simulink model "simulink_model"  (R2015a)
settings: Solver=ode3  StartTime=0.0  StopTime=20  RelTol=1e-3
undefined symbols (not defined in the file or in its folder): MIO, National_Instruments, PCI
libraries: sldrtlib x3, simulink x1
settings Model: SimulationMode=external  ExtModeTrigDuration=30001  Creator=Alunos  LastModifiedBy=Alunos
settings HardwareCC: ProdIntDivRoundTo=Zero  ProdEndianess=LittleEndian  ProdHWDeviceType=Intel->x86/Pentium  TargetIntDivRoundTo=Zero  TargetEndianess=LittleEndian  TargetHWDeviceType=Intel->x86/Pentium
settings RTWCC: SystemTargetFile=rtwin.tlc  TemplateMakefile=rtwin.tmf  Description=Simulink Desktop Real-Time  RTWCompilerOptimization=on
settings CodeAppCC: MaxIdLength=95
settings RTWinTargetCC: TargetPreCompLibLocation=C:\Program Files\MATLAB\R2015a\toolbox\sldrt\lib\win32

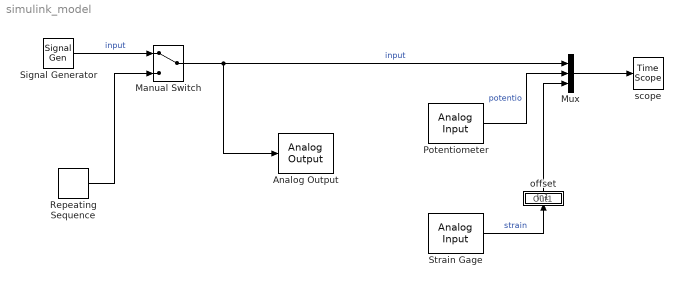
== system simulink_model ==
  Analog Output : sldrtlib/Analog Output  SampleTime=0.001  MaxMissedTicks=10  ShowMissedTicks=off  YieldWhenWaiting=off  DrvName=National_Instruments/PCI-MIO-16E-4  DrvAddress=4294967295  DrvOptions=[0 0 0 0 0 0]  Channels=1  RangeMode=1  VoltRange=1  InitialValue=0  FinalValue=0
      settings: AttributesFormatString=National Instruments\nPCI-MIO-16E-4 [auto]
  Manual Switch : ManualSwitch
  Mux : Mux  Inputs=3
  Potentiometer : sldrtlib/Analog Input  SampleTime=0.001  MaxMissedTicks=10  ShowMissedTicks=off  YieldWhenWaiting=off  DrvName=National_Instruments/PCI-MIO-16E-4  DrvAddress=4294967295  DrvOptions=[0 0 0 0 0 0]  Channels=1  RangeMode=1  VoltRange=1  DataType=1
      settings: AttributesFormatString=National Instruments\nPCI-MIO-16E-4 [auto]
  Repeating Sequence : simulink/Sources/Repeating Sequence  rep_seq_t=[0 0.9999 1 1.9999 2 2.9999 3 4]  rep_seq_y=[1 1 0 0 -1 -1 0 0]
  Signal Generator : SignalGenerator  WaveForm=square
  Strain Gage : sldrtlib/Analog Input  SampleTime=0.001  MaxMissedTicks=10  ShowMissedTicks=off  YieldWhenWaiting=off  DrvName=National_Instruments/PCI-MIO-16E-4  DrvAddress=4294967295  DrvOptions=[0 0 0 0 0 0]  Channels=2  RangeMode=1  VoltRange=1  DataType=1
      settings: AttributesFormatString=National Instruments\nPCI-MIO-16E-4 [auto]
  offset : Subsystem
  scope : TimeScope
  wires:
  Mux/1 -> scope/1
  Potentiometer/1 -> Mux/2  "potentio"
  Signal Generator/1 -> Manual Switch/1  "input"
  Manual Switch/1 -> Analog Output/1, Mux/1  "input"
  Repeating Sequence/1 -> Manual Switch/2
  Strain Gage/1 -> offset/1(In1)  "strain"
  offset/1(Out1) -> Mux/3

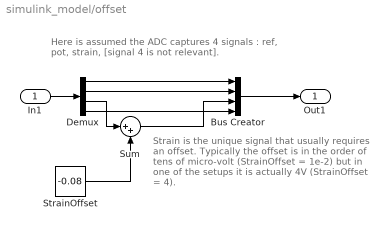
== system simulink_model/offset ==
  note: Strain is the unique signal that usually requires an offset. Typically the offset is in the order of tens of micro-volt (StrainOffset = 1e-2) but in one of the setups it is actually 4V (StrainOffset = 4).
  note: Here is assumed the ADC captures 4 signals :
      | ref, pot, strain, [signal 4 is not relevant].
  In1 : Inport
  Bus Creator : BusCreator
  Demux : Demux
  StrainOffset : Constant  Value=-0.08
  Sum : Sum  Inputs=|++
  Out1 : Outport
  wires:
  In1/1 -> Demux/1
  Bus Creator/1 -> Out1/1
  Demux/1 -> Bus Creator/1
  Demux/2 -> Bus Creator/2
  Demux/4 -> Bus Creator/4
  Demux/3 -> Sum/1
  Sum/1 -> Bus Creator/3
  StrainOffset/1 -> Sum/2
